simulink model "StateFeedbackTest1"  (R2018b)
settings: Solver=VariableStepAuto  StartTime=0.0  StopTime=90  RelTol=1e-3
settings Model: Creator=mmbio  LastModifiedBy=mmbio

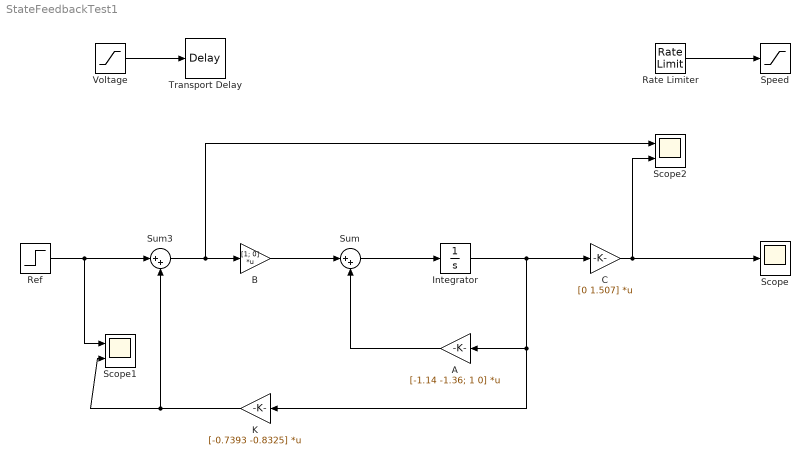
== system StateFeedbackTest1 ==
  A : Gain  Gain=[-1.14 -1.36; 1 0]  Multiplication=Matrix(K*u)
  B : Gain  Gain=[1; 0]  Multiplication=Matrix(K*u)
  C : Gain  Gain=[0 1.507]  Multiplication=Matrix(K*u)
  Integrator : Integrator
  K : Gain  Gain=[-0.7393 -0.8325]  Multiplication=Matrix(K*u)
  Rate Limiter : RateLimiter  RisingSlewLimit=0.65  FallingSlewLimit=-0.65  SampleTimeMode=inherited
  Ref : Step  SampleTime=0
  Scope : Scope
  Scope1 : Scope  NumInputPorts=2
  Scope2 : Scope  NumInputPorts=2
  Speed : Saturate  UpperLimit=1000  LowerLimit=0
  Sum : Sum  Inputs=|++
  Sum3 : Sum  Inputs=|++
  Transport Delay : TransportDelay  DelayTime=0.45
  Voltage : Saturate  UpperLimit=5  LowerLimit=0
  wires:
  Integrator/1 -> K/1, A/1, C/1
  Voltage/1 -> Transport Delay/1
  Rate Limiter/1 -> Speed/1
  K/1 -> Scope1/2, Sum3/2
  Sum/1 -> Integrator/1
  A/1 -> Sum/2
  B/1 -> Sum/1
  Ref/1 -> Scope1/1, Sum3/1
  Sum3/1 -> Scope2/1, B/1
  C/1 -> Scope2/2, Scope/1
